simulink model "CRITIS_1_full"  (R2022b)
settings: Solver=VariableStepAuto  StartTime=0.0  StopTime=7  RelTol=1e-3
(part 2 of 13)

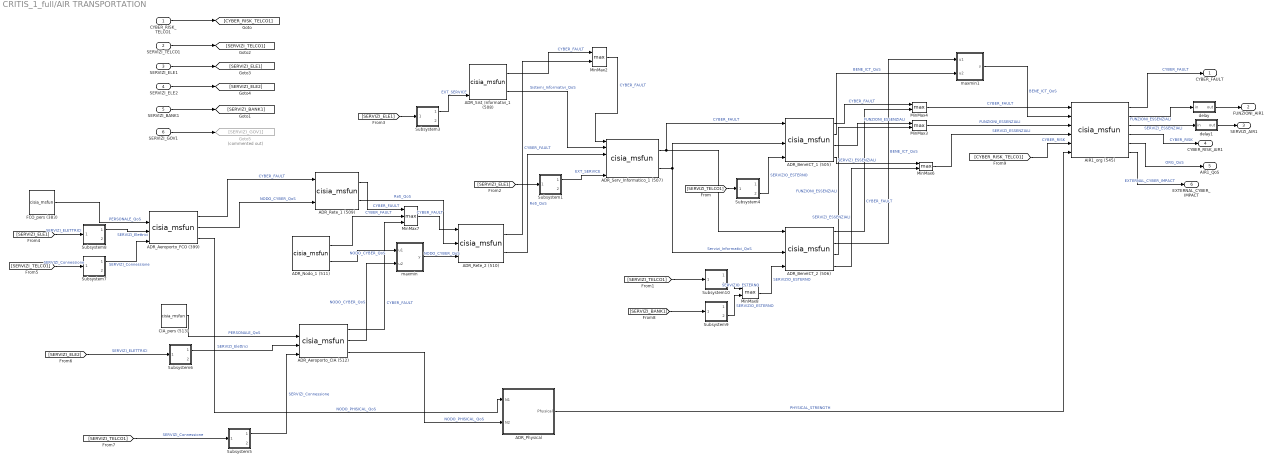
== system CRITIS_1_full/AIR TRANSPORTATION ==
  CYBER_RISK_TELCO1 : Inport
  SERVIZI_TELCO1 : Inport  Port=2
  SERVIZI_ELE1 : Inport  Port=3
  SERVIZI_ELE2 : Inport  Port=4
  SERVIZI_BANK1 : Inport  Port=5
  SERVIZI_GOV1 : Inport  Port=6
  ADR_Aeroporto_CIA (512) : M-S-Function  FunctionName=cisia_msfun  Parameters=Parameter1, Parameter2, Parameter3, resources, Parameter10, codeupdate, step_received, step_computed, dynamic_computed, step_sended, id_entity, id_project, id_type, name_type, color  mask(S-function:msfcn_unit_delay){Parameter1='ADR_Aeroporto_CIA', Parameter2=1, Parameter3='Iside', resources=|, Parameter10=off, codeupdate=off, step_received=|, step_computed=, dynamic_computed=, step_sended=|, id_entity=512, id_project=14, id_type=98, name_type=Nodo_Aeroporto, color=#FFFFFF}
      mask resources=|
      | *** INPUT RESOURCES ***
      | NUM_INPUTS 4
      | CYBER_FAULT (25)
      | PERSONALE_QoS (1)
      | SERVIZI_Elettrici (1)
      | SERVIZI_Connessione (1)
      |
      | *** STATE VARIABLES ***
      | NUM_VARIABLES 38
      | Operative_Level(NUMERIC)(1)(1)
      | Dos_attack(NUMERIC)(1)(0)
      | MITM_attack(NUMERIC)(1)(0)
      | Virus_Attack(NUMERIC)(1)(0)
      | Port_Scan_Attack(NUMERIC)(1)(0)
      | Cyber_Fault(NUMERIC_ARRAY)(25)(0  0  0  0  0  0  0  0  0  0  0  0  0  0  0  0  0  0  0  0  0  0  0  0  0)
      | BGP_hijacking(NUMERIC)(1)(0)
      | Mechanical_Fault(NUMERIC)(1)(0)
      | Power_Fault(NUMERIC)(1)(0)
      | Flooding_Fault(NUMERIC)(1)(0)
      | Fire_Fault(NUMERIC)(1)(0)
      | Unauthorized_Access(NUMERIC)(1)(0)
      | Conn_Fault(NUMERIC)(1)(0)
      | Service_Fault(NUMERIC)(1)(0)
      | BotNet_Attack(NUMERIC)(1)(0)
      | Data_Corruption(NUMERIC)(1)(0)
      | Rouge_Access(NUMERIC)(1)(0)
      | syslog_adm_login(NUMERIC)(1)(0)
      | SW_Change(NUMERIC)(1)(0)
      | Config_Change(NUMERIC)(1)(0)
      | Port_Saturation(NUMERIC)(1)(0)
      | Congestion_Fault(NUMERIC)(1)(0)
      | Perimeter_Security_Fault(NUMERIC)(1)(0)
      | Earthquake_Fault(NUMERIC)(1)(0)
      | Physical_Fault(NUMERIC)(1)(0)
      | Route_Poisoning(NUMERIC)(1)(0)
      | Interface_Down(NUMERIC)(1)(0)
      | Port_Isolation(NUMERIC)(1)(0)
      | Unknown_Device(NUMERIC)(1)(0)
      | USB_Device_Insertion(NUMERIC)(1)(0)
      | TLC_Fault(NUMERIC)(1)(0)
      | SW_Fault(NUMERIC)(1)(0)
      | Internal_Cyber_Risk(NUMERIC)(1)(0)
      | Data_Breach(NUMERIC)(1)(0)
      | Ransomware(NUMERIC)(1)(0)
      | Op_Level2(NUMERIC_ARRAY)(2)(0  0)
      | Possibility_Value(NUMERIC)(1)(0)
      | Necessity_Value(NUMERIC)(1)(0)
      |
      | *** OUTPUT RESOURCES ***
      | NUM_OUTPUTS 3
      | CYBER_FAULT (25)
      | NODO_CYBER_QoS (2)
      | NODO_PHISICAL_QoS (1)
      mask step_received=|
      | cyber_event=zeros(1,25);
      | cyber_event(1)=Dos_attack;
      | cyber_event(2)=MITM_attack;
      | cyber_event(3)=Virus_Attack;
      | cyber_event(4)=Port_Scan_Attack;
      | cyber_event(5)=BGP_hijacking;
      | cyber_event(6)=BotNet_Attack;
      | cyber_event(7)=Data_Corruption;
      | cyber_event(8)=SW_Change;
      | cyber_event(9)=Config_Change;
      | cyber_event(10)=Port_Saturation;
      | cyber_event(11)=Data_Breach;
      | cyber_event(12)=Unauthorized_Access;
      | cyber_event(13)=Unknown_Device;
      | cyber_event(14)=Congestion_Fault;
      | cyber_event(15)=Interface_Down;
      | cyber_event(16)=Port_Isolation;
      | cyber_event(17)=Rouge_Access;
      | cyber_event(18)=Route_Poisoning;
      | cyber_event(19)=SW_Fault;
      | cyber_event(20)=syslog_adm_login;
      | cyber_event(21)=USB_Device_Insertion;
      | cyber_event(22)=Ransomware;
      | cyber_event(23)=0;
      | cyber_event(24)=0;
      | cyber_event(25)=0;
      |
      | Cyber_Fault=max(CYBER_FAULT, transpose(cyber_event));
      |
      | TLC_Fault = 1 - SERVIZI_Connessione;
      | Power_Fault = 1-SERVIZI_Elettrici;
      |
      | Physical_Fault = max([Earthquake_Fault Fire_Fault Flooding_Fault Mechanical_Fault]);
      | Service_Fault = 1 - PERSONALE_QoS;
      |
      | Conn_Fault=max([(1-SERVIZI_Elettrici) (1-SERVIZI_Connessione)]);
      |
      | Operative_Level = (1-TLC_Fault)*(1-max(Cyber_Fault)*0.5)*(1-Physical_Fault)*(1-Power_Fault)*(1-Service_Fault);
      |
      | % Il primo elemento rappersenta possibility e si combima
      | % con il max in quanto rende conto del caso migliore
      | % (perche OL)
      |
      | Op_Level2(1)=  min([1-0.3*max(Cyber_Fault) 1-TLC_Fault 1-Power_Fault 1-Physical_Fault 1-Service_Fault]);
      |
      | % Il secondo elemento rappersenta necessity e si combima
      | % con il min in quanto rende conto del caso peggiore
      | % (perche OL)
      |
      | Op_Level2(2)= min([1-0.6*max(Cyber_Fault) 1-TLC_Fault 1-Power_Fault 1-Physical_Fault 1-Service_Fault]);
      |
      | Possibility_Value = Op_Level2(1);
      | Necessity_Value = Op_Level2(2);
      mask step_sended=|
      | CYBER_FAULT = Cyber_Fault;
      | % NODO_CYBER_QoS=(1-max(Cyber_Fault))*(1-Conn_Fault*0.5);
      | NODO_CYBER_QoS = Op_Level2;
      | NODO_PHISICAL_QoS=1-Physical_Fault;
      mask prompts: Parameter1 "entity name"; Parameter2 "sampling time"; Parameter3 "project"; resources "input resources and state variables"; Parameter10 "Bring state variables to output"; codeupdate "update code from mask"
      mask help: This is a level-2 MATLAB file S-function which demonstrates CISIA entity
      mask DialogControl Container1 Prompt: All parameters
      mask Display: disp('Nodo_Aeroporto');port_label('input',1,'\color{yellow}\spadesuit','texmode','on')
  ADR_Aeroporto_FCO (399) : M-S-Function  FunctionName=cisia_msfun  Parameters=Parameter1, Parameter2, Parameter3, resources, Parameter10, codeupdate, step_received, step_computed, dynamic_computed, step_sended, id_entity, id_project, id_type, name_type, color  mask(S-function:msfcn_unit_delay){Parameter1='ADR_Aeroporto_FCO', Parameter2=1, Parameter3='Iside', resources=|, Parameter10=off, codeupdate=off, step_received=|, step_computed=, dynamic_computed=, step_sended=|, id_entity=399, id_project=14, id_type=98, name_type=Nodo_Aeroporto, color=#FFFFFF}
      mask resources=|
      | *** INPUT RESOURCES ***
      | NUM_INPUTS 4
      | CYBER_FAULT (25)
      | PERSONALE_QoS (1)
      | SERVIZI_Elettrici (1)
      | SERVIZI_Connessione (1)
      |
      | *** STATE VARIABLES ***
      | NUM_VARIABLES 38
      | Operative_Level(NUMERIC)(1)(1)
      | Dos_attack(NUMERIC)(1)(0)
      | MITM_attack(NUMERIC)(1)(0)
      | Virus_Attack(NUMERIC)(1)(0)
      | Port_Scan_Attack(NUMERIC)(1)(0)
      | Cyber_Fault(NUMERIC_ARRAY)(25)(0  0  0  0  0  0  0  0  0  0  0  0  0  0  0  0  0  0  0  0  0  0  0  0  0)
      | BGP_hijacking(NUMERIC)(1)(0)
      | Mechanical_Fault(NUMERIC)(1)(0)
      | Power_Fault(NUMERIC)(1)(0)
      | Flooding_Fault(NUMERIC)(1)(0)
      | Fire_Fault(NUMERIC)(1)(0)
      | Unauthorized_Access(NUMERIC)(1)(0)
      | Conn_Fault(NUMERIC)(1)(0)
      | Service_Fault(NUMERIC)(1)(0)
      | BotNet_Attack(NUMERIC)(1)(0)
      | Data_Corruption(NUMERIC)(1)(0)
      | Rouge_Access(NUMERIC)(1)(0)
      | syslog_adm_login(NUMERIC)(1)(0)
      | SW_Change(NUMERIC)(1)(0)
      | Config_Change(NUMERIC)(1)(0)
      | Port_Saturation(NUMERIC)(1)(0)
      | Congestion_Fault(NUMERIC)(1)(0)
      | Perimeter_Security_Fault(NUMERIC)(1)(0)
      | Earthquake_Fault(NUMERIC)(1)(0)
      | Physical_Fault(NUMERIC)(1)(0)
      | Route_Poisoning(NUMERIC)(1)(0)
      | Interface_Down(NUMERIC)(1)(0)
      | Port_Isolation(NUMERIC)(1)(0)
      | Unknown_Device(NUMERIC)(1)(0)
      | USB_Device_Insertion(NUMERIC)(1)(0)
      | TLC_Fault(NUMERIC)(1)(0)
      | SW_Fault(NUMERIC)(1)(0)
      | Internal_Cyber_Risk(NUMERIC)(1)(0)
      | Data_Breach(NUMERIC)(1)(0)
      | Ransomware(NUMERIC)(1)(0)
      | Op_Level2(NUMERIC_ARRAY)(2)(0  0)
      | Possibility_Value(NUMERIC)(1)(0)
      | Necessity_Value(NUMERIC)(1)(0)
      |
      | *** OUTPUT RESOURCES ***
      | NUM_OUTPUTS 3
      | CYBER_FAULT (25)
      | NODO_CYBER_QoS (2)
      | NODO_PHISICAL_QoS (1)
      mask step_received=|
      | cyber_event=zeros(1,25);
      | cyber_event(1)=Dos_attack;
      | cyber_event(2)=MITM_attack;
      | cyber_event(3)=Virus_Attack;
      | cyber_event(4)=Port_Scan_Attack;
      | cyber_event(5)=BGP_hijacking;
      | cyber_event(6)=BotNet_Attack;
      | cyber_event(7)=Data_Corruption;
      | cyber_event(8)=SW_Change;
      | cyber_event(9)=Config_Change;
      | cyber_event(10)=Port_Saturation;
      | cyber_event(11)=Data_Breach;
      | cyber_event(12)=Unauthorized_Access;
      | cyber_event(13)=Unknown_Device;
      | cyber_event(14)=Congestion_Fault;
      | cyber_event(15)=Interface_Down;
      | cyber_event(16)=Port_Isolation;
      | cyber_event(17)=Rouge_Access;
      | cyber_event(18)=Route_Poisoning;
      | cyber_event(19)=SW_Fault;
      | cyber_event(20)=syslog_adm_login;
      | cyber_event(21)=USB_Device_Insertion;
      | cyber_event(22)=Ransomware;
      | cyber_event(23)=0;
      | cyber_event(24)=0;
      | cyber_event(25)=0;
      |
      | Cyber_Fault=max(CYBER_FAULT, transpose(cyber_event));
      |
      | TLC_Fault = 1 - SERVIZI_Connessione;
      | Power_Fault = 1-SERVIZI_Elettrici;
      |
      | Physical_Fault = max([Earthquake_Fault Fire_Fault Flooding_Fault Mechanical_Fault]);
      | Service_Fault = 1 - PERSONALE_QoS;
      |
      | Conn_Fault=max([(1-SERVIZI_Elettrici) (1-SERVIZI_Connessione)]);
      |
      | Operative_Level = (1-TLC_Fault)*(1-max(Cyber_Fault)*0.5)*(1-Physical_Fault)*(1-Power_Fault)*(1-Service_Fault);
      |
      | % Il primo elemento rappersenta possibility e si combima
      | % con il max in quanto rende conto del caso migliore
      | % (perche OL)
      |
      | Op_Level2(1)=  min([1-0.3*max(Cyber_Fault) 1-TLC_Fault 1-Power_Fault 1-Physical_Fault 1-Service_Fault]);
      |
      | % Il secondo elemento rappersenta necessity e si combima
      | % con il min in quanto rende conto del caso peggiore
      | % (perche OL)
      |
      | Op_Level2(2)= min([1-0.6*max(Cyber_Fault) 1-TLC_Fault 1-Power_Fault 1-Physical_Fault 1-Service_Fault]);
      |
      | Possibility_Value = Op_Level2(1);
      | Necessity_Value = Op_Level2(2);
      mask step_sended=|
      | CYBER_FAULT = Cyber_Fault;
      | % NODO_CYBER_QoS=(1-max(Cyber_Fault))*(1-Conn_Fault*0.5);
      | NODO_CYBER_QoS = Op_Level2;
      | NODO_PHISICAL_QoS=1-Physical_Fault;
      mask prompts: Parameter1 "entity name"; Parameter2 "sampling time"; Parameter3 "project"; resources "input resources and state variables"; Parameter10 "Bring state variables to output"; codeupdate "update code from mask"
      mask help: This is a level-2 MATLAB file S-function which demonstrates CISIA entity
      mask DialogControl Container1 Prompt: All parameters
      mask Display: disp('Nodo_Aeroporto');port_label('input',1,'\color{yellow}\spadesuit','texmode','on')
  ADR_BeneICT_1 (505) : M-S-Function  FunctionName=cisia_msfun  Parameters=Parameter1, Parameter2, Parameter3, resources, Parameter10, codeupdate, step_received, step_computed, dynamic_computed, step_sended, id_entity, id_project, id_type, name_type, color  mask(S-function:msfcn_unit_delay){Parameter1='ADR_BeneICT_1', Parameter2=1, Parameter3='Iside', resources=|, Parameter10=off, codeupdate=off, step_received=|, step_computed=, dynamic_computed=, step_sended=|, id_entity=505, id_project=14, id_type=108, name_type=BeneICT, color=#64D413}
      mask resources=|
      | *** INPUT RESOURCES ***
      | NUM_INPUTS 6
      | CYBER_FAULT (25)
      | Sistemi_Informativi_QoS (2)
      | Reti_QoS (2)
      | Servizi_Informatici_QoS (2)
      | BENE_ICT_QoS (2)
      | SERVIZIO_ESTERNO (20)
      |
      | *** STATE VARIABLES ***
      | NUM_VARIABLES 34
      | Operative_Level(NUMERIC)(1)(1)
      | Dos_attack(NUMERIC)(1)(0)
      | MITM_attack(NUMERIC)(1)(0)
      | Virus_Attack(NUMERIC)(1)(0)
      | Port_Scan_Attack(NUMERIC)(1)(0)
      | Cyber_Fault(NUMERIC_ARRAY)(25)(0  0  0  0  0  0  0  0  0  0  0  0  0  0  0  0  0  0  0  0  0  0  0  0  0)
      | BGP_hijacking(NUMERIC)(1)(0)
      | Unauthorized_Access(NUMERIC)(1)(0)
      | Consumed_Services(NUMERIC_ARRAY)(10)(0  0  0  0  0  0  0  0  0  0)
      | Service_Fault(NUMERIC)(1)(0)
      | BotNet_Attack(NUMERIC)(1)(0)
      | Data_Corruption(NUMERIC)(1)(0)
      | Rouge_Access(NUMERIC)(1)(0)
      | syslog_adm_login(NUMERIC)(1)(0)
      | SW_Change(NUMERIC)(1)(0)
      | Config_Change(NUMERIC)(1)(0)
      | Port_Saturation(NUMERIC)(1)(0)
      | Congestion_Fault(NUMERIC)(1)(0)
      | Route_Poisoning(NUMERIC)(1)(0)
      | Interface_Down(NUMERIC)(1)(0)
      | Port_Isolation(NUMERIC)(1)(0)
      | Unknown_Device(NUMERIC)(1)(0)
      | USB_Device_Insertion(NUMERIC)(1)(0)
      | SW_Fault(NUMERIC)(1)(0)
      | Servizi_Essenziali(NUMERIC_ARRAY)(10)(1  0  0  0  0  0  0  0  0  0)
      | Funzioni_Essenziali(NUMERIC_ARRAY)(10)(0  0  0  0  0  0  0  0  0  0)
      | Consumed_Functions(NUMERIC_ARRAY)(10)(0  0  0  0  0  0  0  0  0  0)
      | Internal_Cyber_Risk(NUMERIC)(1)(0)
      | Data_Breach(NUMERIC)(1)(0)
      | availability_fault(NUMERIC)(1)(0)
      | Ransomware(NUMERIC)(1)(0)
      | Op_Level2(NUMERIC_ARRAY)(2)(0  0)
      | Possibility_Value(NUMERIC)(1)(0)
      | Necessity_Value(NUMERIC)(1)(0)
      |
      | *** OUTPUT RESOURCES ***
      | NUM_OUTPUTS 4
      | CYBER_FAULT (25)
      | BENE_ICT_QoS (2)
      | FUNZIONI_ESSENZIALI (10)
      | SERVIZI_ESSENZIALI (10)
      mask step_received=|
      | cyber_event=zeros(1,25);
      | cyber_event(1)=Dos_attack;
      | cyber_event(2)=MITM_attack;
      | cyber_event(3)=Virus_Attack;
      | cyber_event(4)=Port_Scan_Attack;
      | cyber_event(5)=BGP_hijacking;
      | cyber_event(6)=BotNet_Attack;
      | cyber_event(7)=Data_Corruption;
      | cyber_event(8)=SW_Change;
      | cyber_event(9)=Config_Change;
      | cyber_event(10)=Port_Saturation;
      | cyber_event(11)=Data_Breach;
      | cyber_event(12)=Unauthorized_Access;
      | cyber_event(13)=Unknown_Device;
      | cyber_event(14)=Congestion_Fault;
      | cyber_event(15)=Interface_Down;
      | cyber_event(16)=Port_Isolation;
      | cyber_event(17)=Rouge_Access;
      | cyber_event(18)=Route_Poisoning;
      | cyber_event(19)=SW_Fault;
      | cyber_event(20)=syslog_adm_login;
      | cyber_event(21)=USB_Device_Insertion;
      | cyber_event(22)=Ransomware;
      | cyber_event(23)=0;
      | cyber_event(24)=0;
      | cyber_event(25)=0;
      |
      | Cyber_Fault=max(CYBER_FAULT, transpose(cyber_event));
      |
      | Consumed_Services=SERVIZIO_ESTERNO(1:10);
      | Consumed_Functions=SERVIZIO_ESTERNO(11:20);
      |
      | Service_Fault=max(abs(Servizi_Essenziali-Consumed_Services));
      |
      | availability_fault=1-min([(1-0.5*max(Cyber_Fault)) min(Reti_QoS) min(Sistemi_Informativi_QoS) min(Servizi_Informatici_QoS) min(BENE_ICT_QoS)]);
      |
      | Operative_Level=min([(1-0.5*max(Cyber_Fault)) mean(Reti_QoS) mean(Sistemi_Informativi_QoS) mean(Servizi_Informatici_QoS) mean(BENE_ICT_QoS) 1-Service_Fault]);
      |
      | % Il primo elemento rappersenta possibility e si combima
      | % con il max in quanto rende conto del caso migliore
      | % (perche OL)
      |
      | BNICT=BENE_ICT_QoS;
      |
      | Op_Level2(1)=  min([1-0.3*max(Cyber_Fault) max([use_elem(Reti_QoS,1) use_elem(Sistemi_Informativi_QoS,1) use_elem(Servizi_Informatici_QoS,1) use_elem(BENE_ICT_QoS,1)]) 1-Service_Fault]);
      |
      | % Il secondo elemento rappresenta necessity e si combima
      | % con il min in quanto rende conto del caso peggiore
      | % (perche OL)
      |
      |
      |
      | Op_Level2(2)= min([1-0.6*max(Cyber_Fault) min([use_elem(Reti_QoS,2) use_elem(Sistemi_Informativi_QoS,2) use_elem(Servizi_Informatici_QoS,2) use_elem(BENE_ICT_QoS,2)]) 1-Service_Fault]);
      |
      | Possibility_Value = Op_Level2(1);
      | Necessity_Value = Op_Level2(2);
      mask step_sended=|
      | CYBER_FAULT=Cyber_Fault;
      |
      | FUNZIONI_ESSENZIALI=(1-availability_fault)*Funzioni_Essenziali.*Consumed_Functions;
      |
      | SERVIZI_ESSENZIALI=(1-availability_fault)*Servizi_Essenziali.*Consumed_Services;
      |
      | BENE_ICT_QoS=Op_Level2;
      mask prompts: Parameter1 "entity name"; Parameter2 "sampling time"; Parameter3 "project"; resources "input resources and state variables"; Parameter10 "Bring state variables to output"; codeupdate "update code from mask"
      mask help: This is a level-2 MATLAB file S-function which demonstrates CISIA entity
      mask DialogControl Container1 Prompt: All parameters
      mask Display: disp('BeneICT');port_label('input',2,'\color{yellow}\spadesuit','texmode','on');port_label('input',3,'\color{yellow}\spadesuit','texmode','on');port_label('input',5,'\color{yellow}\spadesuit','texmode','on')
  ADR_BeneICT_2 (506) : M-S-Function  FunctionName=cisia_msfun  Parameters=Parameter1, Parameter2, Parameter3, resources, Parameter10, codeupdate, step_received, step_computed, dynamic_computed, step_sended, id_entity, id_project, id_type, name_type, color  mask(S-function:msfcn_unit_delay){Parameter1='ADR_BeneICT_2', Parameter2=1, Parameter3='Iside', resources=|, Parameter10=off, codeupdate=off, step_received=|, step_computed=, dynamic_computed=, step_sended=|, id_entity=506, id_project=14, id_type=108, name_type=BeneICT, color=#64D413}
      mask resources=|
      | *** INPUT RESOURCES ***
      | NUM_INPUTS 6
      | CYBER_FAULT (25)
      | Sistemi_Informativi_QoS (2)
      | Reti_QoS (2)
      | Servizi_Informatici_QoS (2)
      | BENE_ICT_QoS (2)
      | SERVIZIO_ESTERNO (20)
      |
      | *** STATE VARIABLES ***
      | NUM_VARIABLES 34
      | Operative_Level(NUMERIC)(1)(1)
      | Dos_attack(NUMERIC)(1)(0)
      | MITM_attack(NUMERIC)(1)(0)
      | Virus_Attack(NUMERIC)(1)(0)
      | Port_Scan_Attack(NUMERIC)(1)(0)
      | Cyber_Fault(NUMERIC_ARRAY)(25)(0  0  0  0  0  0  0  0  0  0  0  0  0  0  0  0  0  0  0  0  0  0  0  0  0)
      | BGP_hijacking(NUMERIC)(1)(0)
      | Unauthorized_Access(NUMERIC)(1)(0)
      | Consumed_Services(NUMERIC_ARRAY)(10)(0  0  0  0  0  0  0  0  0  0)
      | Service_Fault(NUMERIC)(1)(0)
      | BotNet_Attack(NUMERIC)(1)(0)
      | Data_Corruption(NUMERIC)(1)(0)
      | Rouge_Access(NUMERIC)(1)(0)
      | syslog_adm_login(NUMERIC)(1)(0)
      | SW_Change(NUMERIC)(1)(0)
      | Config_Change(NUMERIC)(1)(0)
      | Port_Saturation(NUMERIC)(1)(0)
      | Congestion_Fault(NUMERIC)(1)(0)
      | Route_Poisoning(NUMERIC)(1)(0)
      | Interface_Down(NUMERIC)(1)(0)
      | Port_Isolation(NUMERIC)(1)(0)
      | Unknown_Device(NUMERIC)(1)(0)
      | USB_Device_Insertion(NUMERIC)(1)(0)
      | SW_Fault(NUMERIC)(1)(0)
      | Servizi_Essenziali(NUMERIC_ARRAY)(10)(0  1  1  0  0  0  0  0  0  0)
      | Funzioni_Essenziali(NUMERIC_ARRAY)(10)(0  0  0  0  0  0  0  0  0  0)
      | Consumed_Functions(NUMERIC_ARRAY)(10)(0  0  0  0  0  0  0  0  0  0)
      | Internal_Cyber_Risk(NUMERIC)(1)(0)
      | Data_Breach(NUMERIC)(1)(0)
      | availability_fault(NUMERIC)(1)(0)
      | Ransomware(NUMERIC)(1)(0)
      | Op_Level2(NUMERIC_ARRAY)(2)(0  0)
      | Possibility_Value(NUMERIC)(1)(0)
      | Necessity_Value(NUMERIC)(1)(0)
      |
      | *** OUTPUT RESOURCES ***
      | NUM_OUTPUTS 4
      | CYBER_FAULT (25)
      | BENE_ICT_QoS (2)
      | FUNZIONI_ESSENZIALI (10)
      | SERVIZI_ESSENZIALI (10)
      mask step_received=|
      | cyber_event=zeros(1,25);
      | cyber_event(1)=Dos_attack;
      | cyber_event(2)=MITM_attack;
      | cyber_event(3)=Virus_Attack;
      | cyber_event(4)=Port_Scan_Attack;
      | cyber_event(5)=BGP_hijacking;
      | cyber_event(6)=BotNet_Attack;
      | cyber_event(7)=Data_Corruption;
      | cyber_event(8)=SW_Change;
      | cyber_event(9)=Config_Change;
      | cyber_event(10)=Port_Saturation;
      | cyber_event(11)=Data_Breach;
      | cyber_event(12)=Unauthorized_Access;
      | cyber_event(13)=Unknown_Device;
      | cyber_event(14)=Congestion_Fault;
      | cyber_event(15)=Interface_Down;
      | cyber_event(16)=Port_Isolation;
      | cyber_event(17)=Rouge_Access;
      | cyber_event(18)=Route_Poisoning;
      | cyber_event(19)=SW_Fault;
      | cyber_event(20)=syslog_adm_login;
      | cyber_event(21)=USB_Device_Insertion;
      | cyber_event(22)=Ransomware;
      | cyber_event(23)=0;
      | cyber_event(24)=0;
      | cyber_event(25)=0;
      |
      | Cyber_Fault=max(CYBER_FAULT, transpose(cyber_event));
      |
      | Consumed_Services=SERVIZIO_ESTERNO(1:10);
      | Consumed_Functions=SERVIZIO_ESTERNO(11:20);
      |
      | Service_Fault=max(abs(Servizi_Essenziali-Consumed_Services));
      |
      | availability_fault=1-min([(1-0.5*max(Cyber_Fault)) min(Reti_QoS) min(Sistemi_Informativi_QoS) min(Servizi_Informatici_QoS) min(BENE_ICT_QoS)]);
      |
      | Operative_Level=min([(1-0.5*max(Cyber_Fault)) mean(Reti_QoS) mean(Sistemi_Informativi_QoS) mean(Servizi_Informatici_QoS) mean(BENE_ICT_QoS) 1-Service_Fault]);
      |
      | % Il primo elemento rappersenta possibility e si combima
      | % con il max in quanto rende conto del caso migliore
      | % (perche OL)
      |
      | BNICT=BENE_ICT_QoS;
      |
      | Op_Level2(1)=  min([1-0.3*max(Cyber_Fault) max([use_elem(Reti_QoS,1) use_elem(Sistemi_Informativi_QoS,1) use_elem(Servizi_Informatici_QoS,1) use_elem(BENE_ICT_QoS,1)]) 1-Service_Fault]);
      |
      | % Il secondo elemento rappresenta necessity e si combima
      | % con il min in quanto rende conto del caso peggiore
      | % (perche OL)
      |
      |
      |
      | Op_Level2(2)= min([1-0.6*max(Cyber_Fault) min([use_elem(Reti_QoS,2) use_elem(Sistemi_Informativi_QoS,2) use_elem(Servizi_Informatici_QoS,2) use_elem(BENE_ICT_QoS,2)]) 1-Service_Fault]);
      |
      | Possibility_Value = Op_Level2(1);
      | Necessity_Value = Op_Level2(2);
      mask step_sended=|
      | CYBER_FAULT=Cyber_Fault;
      |
      | FUNZIONI_ESSENZIALI=(1-availability_fault)*Funzioni_Essenziali.*Consumed_Functions;
      |
      | SERVIZI_ESSENZIALI=(1-availability_fault)*Servizi_Essenziali.*Consumed_Services;
      |
      | BENE_ICT_QoS=Op_Level2;
      mask prompts: Parameter1 "entity name"; Parameter2 "sampling time"; Parameter3 "project"; resources "input resources and state variables"; Parameter10 "Bring state variables to output"; codeupdate "update code from mask"
      mask help: This is a level-2 MATLAB file S-function which demonstrates CISIA entity
      mask DialogControl Container1 Prompt: All parameters
      mask Display: disp('BeneICT');port_label('input',2,'\color{yellow}\spadesuit','texmode','on');port_label('input',3,'\color{yellow}\spadesuit','texmode','on');port_label('input',5,'\color{yellow}\spadesuit','texmode','on')
  ADR_Nodo_1 (511) : M-S-Function  FunctionName=cisia_msfun  Parameters=Parameter1, Parameter2, Parameter3, resources, Parameter10, codeupdate, step_received, step_computed, dynamic_computed, step_sended, id_entity, id_project, id_type, name_type, color  mask(S-function:msfcn_unit_delay){Parameter1='ADR_Nodo_1', Parameter2=1, Parameter3='Iside', resources=|, Parameter10=off, codeupdate=off, step_received=|, step_computed=, dynamic_computed=, step_sended=|, id_entity=511, id_project=14, id_type=109, name_type=Nodo_Datacenter, color=#DCF6F7}
      mask resources=|
      | *** INPUT RESOURCES ***
      | NUM_INPUTS 0
      |
      | *** STATE VARIABLES ***
      | NUM_VARIABLES 32
      | Operative_Level(NUMERIC)(1)(1)
      | Dos_attack(NUMERIC)(1)(0)
      | MITM_attack(NUMERIC)(1)(0)
      | Virus_Attack(NUMERIC)(1)(0)
      | Port_Scan_Attack(NUMERIC)(1)(0)
      | Cyber_Fault(NUMERIC_ARRAY)(25)(0  0  0  0  0  0  0  0  0  0  0  0  0  0  0  0  0  0  0  0  0  0  0  0  0)
      | BGP_hijacking(NUMERIC)(1)(0)
      | Mechanical_Fault(NUMERIC)(1)(0)
      | Unauthorized_Access(NUMERIC)(1)(0)
      | Conn_Fault(NUMERIC)(1)(0)
      | BotNet_Attack(NUMERIC)(1)(0)
      | Data_Corruption(NUMERIC)(1)(0)
      | Rouge_Access(NUMERIC)(1)(0)
      | syslog_adm_login(NUMERIC)(1)(0)
      | SW_Change(NUMERIC)(1)(0)
      | Config_Change(NUMERIC)(1)(0)
      | Port_Saturation(NUMERIC)(1)(0)
      | Congestion_Fault(NUMERIC)(1)(0)
      | Route2(NUMERIC)(1)(0)
      | Route_Poisoning(NUMERIC)(1)(0)
      | Interface_Down(NUMERIC)(1)(0)
      | Port_Isolation(NUMERIC)(1)(0)
      | Unknown_Device(NUMERIC)(1)(0)
      | USB_Device_Insertion(NUMERIC)(1)(0)
      | GEO_localization(STRING)(100)()
      | SW_Fault(NUMERIC)(1)(0)
      | Internal_Cyber_Risk(NUMERIC)(1)(0)
      | Data_Breach(NUMERIC)(1)(0)
      | Ransomware(NUMERIC)(1)(0)
      | Op_Level2(NUMERIC_ARRAY)(2)(0  0)
      | Possibility_Value(NUMERIC)(1)(0)
      | Necessity_Value(NUMERIC)(1)(0)
      |
      | *** OUTPUT RESOURCES ***
      | NUM_OUTPUTS 2
      | CYBER_FAULT (25)
      | NODO_CYBER_QoS (2)
      mask step_received=|
      | cyber_event=zeros(1,25);
      | cyber_event(1)=Dos_attack;
      | cyber_event(2)=MITM_attack;
      | cyber_event(3)=Virus_Attack;
      | cyber_event(4)=Port_Scan_Attack;
      | cyber_event(5)=BGP_hijacking;
      | cyber_event(6)=BotNet_Attack;
      | cyber_event(7)=Data_Corruption;
      | cyber_event(8)=SW_Change;
      | cyber_event(9)=Config_Change;
      | cyber_event(10)=Port_Saturation;
      | cyber_event(11)=Data_Breach;
      | cyber_event(12)=Unauthorized_Access;
      | cyber_event(13)=Unknown_Device;
      | cyber_event(14)=Congestion_Fault;
      | cyber_event(15)=Interface_Down;
      | cyber_event(16)=Port_Isolation;
      | cyber_event(17)=Rouge_Access;
      | cyber_event(18)=Route_Poisoning;
      | cyber_event(19)=SW_Fault;
      | cyber_event(20)=syslog_adm_login;
      | cyber_event(21)=USB_Device_Insertion;
      | cyber_event(22)=Ransomware;
      | cyber_event(23)=0;
      | cyber_event(24)=0;
      | cyber_event(25)=0;
      |
      | Cyber_Fault=transpose(cyber_event);
      |
      | Conn_Fault=max([Dos_attack BGP_hijacking Route_Poisoning Interface_Down Mechanical_Fault] );
      |
      |
      | Operative_Level=min((1-Conn_Fault),(1-0.5*max(Cyber_Fault)));
      |
      | % Il primo elemento rappersenta possibility e si combima
      | % con il max in quanto rende conto del caso migliore
      | % (perche OL)
      |
      | Op_Level2(1)=  min([1-0.3*max(Cyber_Fault) 1-Conn_Fault]);
      |
      | % Il secondo elemento rappersenta necessity e si combima
      | % con il min in quanto rende conto del caso peggiore
      | % (perche OL)
      |
      | Op_Level2(2)= min([1-0.6*max(Cyber_Fault) 1-Conn_Fault]);
      |
      | Possibility_Value = Op_Level2(1);
      | Necessity_Value = Op_Level2(2);
      mask step_sended=|
      | CYBER_FAULT=Cyber_Fault;
      |
      |
      | NODO_CYBER_QoS=Op_Level2;
      mask prompts: Parameter1 "entity name"; Parameter2 "sampling time"; Parameter3 "project"; resources "input resources and state variables"; Parameter10 "Bring state variables to output"; codeupdate "update code from mask"
      mask help: This is a level-2 MATLAB file S-function which demonstrates CISIA entity
      mask DialogControl Container1 Prompt: All parameters
      mask Display: disp('Nodo_Datacenter')
  ADR_Physical : MATLAB Function  TreatAsAtomicUnit=on
  ADR_Rete_1 (509) : M-S-Function  FunctionName=cisia_msfun  Parameters=Parameter1, Parameter2, Parameter3, resources, Parameter10, codeupdate, step_received, step_computed, dynamic_computed, step_sended, id_entity, id_project, id_type, name_type, color  mask(S-function:msfcn_unit_delay){Parameter1='ADR_Rete_1', Parameter2=1, Parameter3='Iside', resources=|, Parameter10=off, codeupdate=off, step_received=|, step_computed=, dynamic_computed=, step_sended=|, id_entity=509, id_project=14, id_type=82, name_type=Reti_Sito, color=#45B5ED}
      mask resources=|
      | *** INPUT RESOURCES ***
      | NUM_INPUTS 3
      | CYBER_FAULT (25)
      | Reti_QoS (2)
      | NODO_CYBER_QoS (2)
      |
      | *** STATE VARIABLES ***
      | NUM_VARIABLES 34
      | Operative_Level(NUMERIC)(1)(1)
      | Dos_attack(NUMERIC)(1)(0)
      | MITM_attack(NUMERIC)(1)(0)
      | Virus_Attack(NUMERIC)(1)(0)
      | Port_Scan_Attack(NUMERIC)(1)(0)
      | Cyber_Fault(NUMERIC_ARRAY)(25)(0  0  0  0  0  0  0  0  0  0  0  0  0  0  0  0  0  0  0  0  0  0  0  0  0)
      | BGP_hijacking(NUMERIC)(1)(0)
      | Mechanical_Fault(NUMERIC)(1)(0)
      | Unauthorized_Access(NUMERIC)(1)(0)
      | Conn_Fault(NUMERIC)(1)(0)
      | BotNet_Attack(NUMERIC)(1)(0)
      | Data_Corruption(NUMERIC)(1)(0)
      | Rouge_Access(NUMERIC)(1)(0)
      | syslog_adm_login(NUMERIC)(1)(0)
      | SW_Change(NUMERIC)(1)(0)
      | Config_Change(NUMERIC)(1)(0)
      | Port_Saturation(NUMERIC)(1)(0)
      | Congestion_Fault(NUMERIC)(1)(0)
      | Physical_Fault(NUMERIC)(1)(0)
      | Route2(NUMERIC)(1)(0)
      | Route_Poisoning(NUMERIC)(1)(0)
      | Interface_Down(NUMERIC)(1)(0)
      | Port_Isolation(NUMERIC)(1)(0)
      | Unknown_Device(NUMERIC)(1)(0)
      | USB_Device_Insertion(NUMERIC)(1)(0)
      | Risorsa(NUMERIC)(1)(0)
      | GEO_localization(STRING)(100)()
      | SW_Fault(NUMERIC)(1)(0)
      | Internal_Cyber_Risk(NUMERIC)(1)(0)
      | Data_Breach(NUMERIC)(1)(0)
      | Ransomware(NUMERIC)(1)(0)
      | Op_Level2(NUMERIC_ARRAY)(2)(0  0)
      | Possibility_Value(NUMERIC)(1)(0)
      | Necessity_Value(NUMERIC)(1)(0)
      |
      | *** OUTPUT RESOURCES ***
      | NUM_OUTPUTS 2
      | CYBER_FAULT (25)
      | Reti_QoS (2)
      mask step_received=|
      | cyber_event=zeros(1,25);
      | cyber_event(1)=Dos_attack;
      | cyber_event(2)=MITM_attack;
      | cyber_event(3)=Virus_Attack;
      | cyber_event(4)=Port_Scan_Attack;
      | cyber_event(5)=BGP_hijacking;
      | cyber_event(6)=BotNet_Attack;
      | cyber_event(7)=Data_Corruption;
      | cyber_event(8)=SW_Change;
      | cyber_event(9)=Config_Change;
      | cyber_event(10)=Port_Saturation;
      | cyber_event(11)=Data_Breach;
      | cyber_event(12)=Unauthorized_Access;
      | cyber_event(13)=Unknown_Device;
      | cyber_event(14)=Congestion_Fault;
      | cyber_event(15)=Interface_Down;
      | cyber_event(16)=Port_Isolation;
      | cyber_event(17)=Rouge_Access;
      | cyber_event(18)=Route_Poisoning;
      | cyber_event(19)=SW_Fault;
      | cyber_event(20)=syslog_adm_login;
      | cyber_event(21)=USB_Device_Insertion;
      | cyber_event(22)=Ransomware;
      | cyber_event(23)=0;
      | cyber_event(24)=0;
      | cyber_event(25)=0;
      |
      | Cyber_Fault=max(CYBER_FAULT, transpose(cyber_event));
      |
      | Conn_Fault=max([Dos_attack BGP_hijacking Route_Poisoning Interface_Down Mechanical_Fault] );
      |
      | Operative_Level=min([(1-Conn_Fault) (1-0.5*max(Cyber_Fault))  mean(Reti_QoS)  mean(NODO_CYBER_QoS)]);
      |
      | % Il primo elemento rappersenta possibility e si combima
      | % con il max in quanto rende conto del caso migliore
      | % (perche OL)
      |
      | Op_Level2(1)=  min([1-0.3*max(Cyber_Fault) max([use_elem(Reti_QoS,1) use_elem(NODO_CYBER_QoS,1)]) 1-Conn_Fault]);
      |
      | % Il secondo elemento rappersenta necessity e si combima
      | % con il min in quanto rende conto del caso peggiore
      | % (perche OL)
      |
      | Op_Level2(2)= min([1-0.6*max(Cyber_Fault) min([use_elem(Reti_QoS,2) use_elem(NODO_CYBER_QoS,2)]) 1-Conn_Fault]);
      |
      | Possibility_Value = Op_Level2(1);
      | Necessity_Value = Op_Level2(2);
      mask step_sended=|
      | CYBER_FAULT=Cyber_Fault;
      |
      |
      | Reti_QoS=Op_Level2;
      mask prompts: Parameter1 "entity name"; Parameter2 "sampling time"; Parameter3 "project"; resources "input resources and state variables"; Parameter10 "Bring state variables to output"; codeupdate "update code from mask"
      mask help: This is a level-2 MATLAB file S-function which demonstrates CISIA entity
      mask DialogControl Container1 Prompt: All parameters
      mask Display: disp('Reti_Sito');port_label('input',2,'\color{yellow}\spadesuit','texmode','on')
  ADR_Rete_2 (510) : M-S-Function  FunctionName=cisia_msfun  Parameters=Parameter1, Parameter2, Parameter3, resources, Parameter10, codeupdate, step_received, step_computed, dynamic_computed, step_sended, id_entity, id_project, id_type, name_type, color  mask(S-function:msfcn_unit_delay){Parameter1='ADR_Rete_2', Parameter2=1, Parameter3='Iside', resources=|, Parameter10=off, codeupdate=off, step_received=|, step_computed=, dynamic_computed=, step_sended=|, id_entity=510, id_project=14, id_type=82, name_type=Reti_Sito, color=#45B5ED}
      mask resources=|
      | *** INPUT RESOURCES ***
      | NUM_INPUTS 3
      | CYBER_FAULT (25)
      | Reti_QoS (2)
      | NODO_CYBER_QoS (2)
      |
      | *** STATE VARIABLES ***
      | NUM_VARIABLES 34
      | Operative_Level(NUMERIC)(1)(1)
      | Dos_attack(NUMERIC)(1)(0)
      | MITM_attack(NUMERIC)(1)(0)
      | Virus_Attack(NUMERIC)(1)(0)
      | Port_Scan_Attack(NUMERIC)(1)(0)
      | Cyber_Fault(NUMERIC_ARRAY)(25)(0  0  0  0  0  0  0  0  0  0  0  0  0  0  0  0  0  0  0  0  0  0  0  0  0)
      | BGP_hijacking(NUMERIC)(1)(0)
      | Mechanical_Fault(NUMERIC)(1)(0)
      | Unauthorized_Access(NUMERIC)(1)(0)
      | Conn_Fault(NUMERIC)(1)(0)
      | BotNet_Attack(NUMERIC)(1)(0)
      | Data_Corruption(NUMERIC)(1)(0)
      | Rouge_Access(NUMERIC)(1)(0)
      | syslog_adm_login(NUMERIC)(1)(0)
      | SW_Change(NUMERIC)(1)(0)
      | Config_Change(NUMERIC)(1)(0)
      | Port_Saturation(NUMERIC)(1)(0)
      | Congestion_Fault(NUMERIC)(1)(0)
      | Physical_Fault(NUMERIC)(1)(0)
      | Route2(NUMERIC)(1)(0)
      | Route_Poisoning(NUMERIC)(1)(0)
      | Interface_Down(NUMERIC)(1)(0)
      | Port_Isolation(NUMERIC)(1)(0)
      | Unknown_Device(NUMERIC)(1)(0)
      | USB_Device_Insertion(NUMERIC)(1)(0)
      | Risorsa(NUMERIC)(1)(0)
      | GEO_localization(STRING)(100)()
      | SW_Fault(NUMERIC)(1)(0)
      | Internal_Cyber_Risk(NUMERIC)(1)(0)
      | Data_Breach(NUMERIC)(1)(0)
      | Ransomware(NUMERIC)(1)(0)
      | Op_Level2(NUMERIC_ARRAY)(2)(0  0)
      | Possibility_Value(NUMERIC)(1)(0)
      | Necessity_Value(NUMERIC)(1)(0)
      |
      | *** OUTPUT RESOURCES ***
      | NUM_OUTPUTS 2
      | CYBER_FAULT (25)
      | Reti_QoS (2)
      mask step_received=|
      | cyber_event=zeros(1,25);
      | cyber_event(1)=Dos_attack;
      | cyber_event(2)=MITM_attack;
      | cyber_event(3)=Virus_Attack;
      | cyber_event(4)=Port_Scan_Attack;
      | cyber_event(5)=BGP_hijacking;
      | cyber_event(6)=BotNet_Attack;
      | cyber_event(7)=Data_Corruption;
      | cyber_event(8)=SW_Change;
      | cyber_event(9)=Config_Change;
      | cyber_event(10)=Port_Saturation;
      | cyber_event(11)=Data_Breach;
      | cyber_event(12)=Unauthorized_Access;
      | cyber_event(13)=Unknown_Device;
      | cyber_event(14)=Congestion_Fault;
      | cyber_event(15)=Interface_Down;
      | cyber_event(16)=Port_Isolation;
      | cyber_event(17)=Rouge_Access;
      | cyber_event(18)=Route_Poisoning;
      | cyber_event(19)=SW_Fault;
      | cyber_event(20)=syslog_adm_login;
      | cyber_event(21)=USB_Device_Insertion;
      | cyber_event(22)=Ransomware;
      | cyber_event(23)=0;
      | cyber_event(24)=0;
      | cyber_event(25)=0;
      |
      | Cyber_Fault=max(CYBER_FAULT, transpose(cyber_event));
      |
      | Conn_Fault=max([Dos_attack BGP_hijacking Route_Poisoning Interface_Down Mechanical_Fault] );
      |
      | Operative_Level=min([(1-Conn_Fault) (1-0.5*max(Cyber_Fault))  mean(Reti_QoS)  mean(NODO_CYBER_QoS)]);
      |
      | % Il primo elemento rappersenta possibility e si combima
      | % con il max in quanto rende conto del caso migliore
      | % (perche OL)
      |
      | Op_Level2(1)=  min([1-0.3*max(Cyber_Fault) max([use_elem(Reti_QoS,1) use_elem(NODO_CYBER_QoS,1)]) 1-Conn_Fault]);
      |
      | % Il secondo elemento rappersenta necessity e si combima
      | % con il min in quanto rende conto del caso peggiore
      | % (perche OL)
      |
      | Op_Level2(2)= min([1-0.6*max(Cyber_Fault) min([use_elem(Reti_QoS,2) use_elem(NODO_CYBER_QoS,2)]) 1-Conn_Fault]);
      |
      | Possibility_Value = Op_Level2(1);
      | Necessity_Value = Op_Level2(2);
      mask step_sended=|
      | CYBER_FAULT=Cyber_Fault;
      |
      |
      | Reti_QoS=Op_Level2;
      mask prompts: Parameter1 "entity name"; Parameter2 "sampling time"; Parameter3 "project"; resources "input resources and state variables"; Parameter10 "Bring state variables to output"; codeupdate "update code from mask"
      mask help: This is a level-2 MATLAB file S-function which demonstrates CISIA entity
      mask DialogControl Container1 Prompt: All parameters
      mask Display: disp('Reti_Sito')
  ADR_Serv_Informatico_1 (507) : M-S-Function  FunctionName=cisia_msfun  Parameters=Parameter1, Parameter2, Parameter3, resources, Parameter10, codeupdate, step_received, step_computed, dynamic_computed, step_sended, id_entity, id_project, id_type, name_type, color  mask(S-function:msfcn_unit_delay){Parameter1='ADR_Serv_Informatico_1', Parameter2=1, Parameter3='Iside', resources=|, Parameter10=off, codeupdate=off, step_received=|, step_computed=, dynamic_computed=, step_sended=|, id_entity=507, id_project=14, id_type=83, name_type=Servizi_Informatici, color=#6FD0E8}
      mask resources=|
      | *** INPUT RESOURCES ***
      | NUM_INPUTS 6
      | CYBER_FAULT (25)
      | Sistemi_Informativi_QoS (2)
      | Reti_QoS (2)
      | Servizi_Informatici_QoS (2)
      | BENE_ICT_QoS (2)
      | EXT_SERVICE (1)
      |
      | *** STATE VARIABLES ***
      | NUM_VARIABLES 31
      | Operative_Level(NUMERIC)(1)(1)
      | Dos_attack(NUMERIC)(1)(0)
      | MITM_attack(NUMERIC)(1)(0)
      | Virus_Attack(NUMERIC)(1)(0)
      | Port_Scan_Attack(NUMERIC)(1)(0)
      | Cyber_Fault(NUMERIC_ARRAY)(25)(0  0  0  0  0  0  0  0  0  0  0  0  0  0  0  0  0  0  0  0  0  0  0  0  0)
      | BGP_hijacking(NUMERIC)(1)(0)
      | Mechanical_Fault(NUMERIC)(1)(0)
      | Unauthorized_Access(NUMERIC)(1)(0)
      | Service_Fault(NUMERIC)(1)(0)
      | BotNet_Attack(NUMERIC)(1)(0)
      | Data_Corruption(NUMERIC)(1)(0)
      | Rouge_Access(NUMERIC)(1)(0)
      | syslog_adm_login(NUMERIC)(1)(0)
      | SW_Change(NUMERIC)(1)(0)
      | Config_Change(NUMERIC)(1)(0)
      | Port_Saturation(NUMERIC)(1)(0)
      | Congestion_Fault(NUMERIC)(1)(0)
      | Route2(NUMERIC)(1)(0)
      | Route_Poisoning(NUMERIC)(1)(0)
      | Interface_Down(NUMERIC)(1)(0)
      | Port_Isolation(NUMERIC)(1)(0)
      | Unknown_Device(NUMERIC)(1)(0)
      | USB_Device_Insertion(NUMERIC)(1)(0)
      | SW_Fault(NUMERIC)(1)(0)
      | Internal_Cyber_Risk(NUMERIC)(1)(0)
      | Data_Breach(NUMERIC)(1)(0)
      | Ransomware(NUMERIC)(1)(0)
      | Op_Level2(NUMERIC_ARRAY)(2)(0  0)
      | Possibility_Value(NUMERIC)(1)(0)
      | Necessity_Value(NUMERIC)(1)(0)
      |
      | *** OUTPUT RESOURCES ***
      | NUM_OUTPUTS 2
      | CYBER_FAULT (25)
      | Servizi_Informatici_QoS (2)
      mask step_received=|
      | cyber_event=zeros(1,25);
      | cyber_event(1)=Dos_attack;
      | cyber_event(2)=MITM_attack;
      | cyber_event(3)=Virus_Attack;
      | cyber_event(4)=Port_Scan_Attack;
      | cyber_event(5)=BGP_hijacking;
      | cyber_event(6)=BotNet_Attack;
      | cyber_event(7)=Data_Corruption;
      | cyber_event(8)=SW_Change;
      | cyber_event(9)=Config_Change;
      | cyber_event(10)=Port_Saturation;
      | cyber_event(11)=Data_Breach;
      | cyber_event(12)=Unauthorized_Access;
      | cyber_event(13)=Unknown_Device;
      | cyber_event(14)=Congestion_Fault;
      | cyber_event(15)=Interface_Down;
      | cyber_event(16)=Port_Isolation;
      | cyber_event(17)=Rouge_Access;
      | cyber_event(18)=Route_Poisoning;
      | cyber_event(19)=SW_Fault;
      | cyber_event(20)=syslog_adm_login;
      | cyber_event(21)=USB_Device_Insertion;
      | cyber_event(22)=Ransomware;
      | cyber_event(23)=0;
      | cyber_event(24)=0;
      | cyber_event(25)=0;
      |
      | Cyber_Fault=max(CYBER_FAULT, transpose(cyber_event));
      |
      | SW_Fault=max([Virus_Attack Data_Corruption SW_Change] );
      |
      | Service_Fault=1-EXT_SERVICE;
      |
      | Operative_Level=min([(1-Service_Fault) (1-SW_Fault) (1- 0.5 * max(Cyber_Fault))  mean(Reti_QoS)  mean(Sistemi_Informativi_QoS) mean(Servizi_Informatici_QoS)  mean(BENE_ICT_QoS)]);
      |
      | % Il primo elemento rappersenta possibility e si combima
      | % con il max in quanto rende conto del caso migliore
      | % (perche OL)
      |
      | Op_Level2(1)=  min([1-0.3*max(Cyber_Fault) max([use_elem(Reti_QoS,1) use_elem(Sistemi_Informativi_QoS,1) use_elem(Servizi_Informatici_QoS,1) use_elem(BENE_ICT_QoS,1)]) 1-Service_Fault (1-SW_Fault)]);
      |
      | % Il secondo elemento rappersenta necessity e si combima
      | % con il min in quanto rende conto del caso peggiore
      | % (perche OL)
      |
      | Op_Level2(2)= min([1-0.6*max(Cyber_Fault) min([use_elem(Reti_QoS,2) use_elem(Sistemi_Informativi_QoS,2) use_elem(Servizi_Informatici_QoS,2) use_elem(BENE_ICT_QoS,2)]) 1-Service_Fault 1-SW_Fault]);
      |
      | Possibility_Value = Op_Level2(1);
      | Necessity_Value = Op_Level2(2);
      mask step_sended=|
      | CYBER_FAULT=Cyber_Fault;
      |
      | Servizi_Informatici_QoS=Op_Level2;
      mask prompts: Parameter1 "entity name"; Parameter2 "sampling time"; Parameter3 "project"; resources "input resources and state variables"; Parameter10 "Bring state variables to output"; codeupdate "update code from mask"
      mask help: This is a level-2 MATLAB file S-function which demonstrates CISIA entity
      mask DialogControl Container1 Prompt: All parameters
      mask Display: disp('Servizi_Informatici');port_label('input',4,'\color{yellow}\spadesuit','texmode','on');port_label('input',5,'\color{yellow}\spadesuit','texmode','on')
  ADR_Sist_Informativi_1 (508) : M-S-Function  FunctionName=cisia_msfun  Parameters=Parameter1, Parameter2, Parameter3, resources, Parameter10, codeupdate, step_received, step_computed, dynamic_computed, step_sended, id_entity, id_project, id_type, name_type, color  mask(S-function:msfcn_unit_delay){Parameter1='ADR_Sist_Informativi_1', Parameter2=1, Parameter3='Iside', resources=|, Parameter10=off, codeupdate=off, step_received=|, step_computed=, dynamic_computed=, step_sended=|, id_entity=508, id_project=14, id_type=81, name_type=Sistemi_Informativi, color=#59F2F7}
      mask resources=|
      | *** INPUT RESOURCES ***
      | NUM_INPUTS 5
      | CYBER_FAULT (25)
      | Sistemi_Informativi_QoS (2)
      | Reti_QoS (2)
      | Servizi_Informatici_QoS (2)
      | EXT_SERVICE (1)
      |
      | *** STATE VARIABLES ***
      | NUM_VARIABLES 33
      | Operative_Level(NUMERIC)(1)(1)
      | Dos_attack(NUMERIC)(1)(0)
      | MITM_attack(NUMERIC)(1)(0)
      | Virus_Attack(NUMERIC)(1)(0)
      | Port_Scan_Attack(NUMERIC)(1)(0)
      | Cyber_Fault(NUMERIC_ARRAY)(25)(0  0  0  0  0  0  0  0  0  0  0  0  0  0  0  0  0  0  0  0  0  0  0  0  0)
      | BGP_hijacking(NUMERIC)(1)(0)
      | Mechanical_Fault(NUMERIC)(1)(0)
      | Power_Fault(NUMERIC)(1)(0)
      | Unauthorized_Access(NUMERIC)(1)(0)
      | Consumed_Services(NUMERIC_ARRAY)(10)(0  0  0  0  0  0  0  0  0  0)
      | Service_Fault(NUMERIC)(1)(0)
      | BotNet_Attack(NUMERIC)(1)(0)
      | Data_Corruption(NUMERIC)(1)(0)
      | Rouge_Access(NUMERIC)(1)(0)
      | syslog_adm_login(NUMERIC)(1)(0)
      | SW_Change(NUMERIC)(1)(0)
      | Config_Change(NUMERIC)(1)(0)
      | Port_Saturation(NUMERIC)(1)(0)
      | Congestion_Fault(NUMERIC)(1)(0)
      | Route_Poisoning(NUMERIC)(1)(0)
      | Interface_Down(NUMERIC)(1)(0)
      | Port_Isolation(NUMERIC)(1)(0)
      | Unknown_Device(NUMERIC)(1)(0)
      | USB_Device_Insertion(NUMERIC)(1)(0)
      | Computational_Fault(NUMERIC)(1)(0)
      | SW_Fault(NUMERIC)(1)(0)
      | Internal_Cyber_Risk(NUMERIC)(1)(0)
      | Data_Breach(NUMERIC)(1)(0)
      | Ransomware(NUMERIC)(1)(0)
      | Op_Level2(NUMERIC_ARRAY)(2)(0  0)
      | Possibility_Value(NUMERIC)(1)(0)
      | Necessity_Value(NUMERIC)(1)(0)
      |
      | *** OUTPUT RESOURCES ***
      | NUM_OUTPUTS 2
      | CYBER_FAULT (25)
      | Sistemi_Informativi_QoS (2)
      mask step_received=|
      | cyber_event=zeros(1,25);
      | cyber_event(1)=Dos_attack;
      | cyber_event(2)=MITM_attack;
      | cyber_event(3)=Virus_Attack;
      | cyber_event(4)=Port_Scan_Attack;
      | cyber_event(5)=BGP_hijacking;
      | cyber_event(6)=BotNet_Attack;
      | cyber_event(7)=Data_Corruption;
      | cyber_event(8)=SW_Change;
      | cyber_event(9)=Config_Change;
      | cyber_event(10)=Port_Saturation;
      | cyber_event(11)=Data_Breach;
      | cyber_event(12)=Unauthorized_Access;
      | cyber_event(13)=Unknown_Device;
      | cyber_event(14)=Congestion_Fault;
      | cyber_event(15)=Interface_Down;
      | cyber_event(16)=Port_Isolation;
      | cyber_event(17)=Rouge_Access;
      | cyber_event(18)=Route_Poisoning;
      | cyber_event(19)=SW_Fault;
      | cyber_event(20)=syslog_adm_login;
      | cyber_event(21)=USB_Device_Insertion;
      | cyber_event(22)=Ransomware;
      | cyber_event(23)=0;
      | cyber_event(24)=0;
      | cyber_event(25)=0;
      |
      | Cyber_Fault=max(CYBER_FAULT, transpose(cyber_event));
      |
      | Computational_Fault=max([Dos_attack Virus_Attack BotNet_Attack Config_Change Mechanical_Fault] );
      |
      | Service_Fault=1-EXT_SERVICE;
      |
      | Operative_Level=min([(1-Service_Fault) (1-Computational_Fault) (1-0.5*max(Cyber_Fault))  mean(Reti_QoS)  mean(Sistemi_Informativi_QoS)  mean(Servizi_Informatici_QoS)]);
      |
      | % Il primo elemento rappersenta possibility e si combima
      | % con il max in quanto rende conto del caso migliore
      | % (perche OL)
      |
      | Op_Level2(1)=  min([1-0.3*max(Cyber_Fault) max([use_elem(Reti_QoS,1) use_elem(Sistemi_Informativi_QoS,1) use_elem(Servizi_Informatici_QoS,1)]) 1-Service_Fault (1-Computational_Fault)]);
      |
      | % Il secondo elemento rappersenta necessity e si combima
      | % con il min in quanto rende conto del caso peggiore
      | % (perche OL)
      |
      | Op_Level2(2)= min([1-0.6*max(Cyber_Fault) min([use_elem(Reti_QoS,2) use_elem(Sistemi_Informativi_QoS,2) use_elem(Servizi_Informatici_QoS,2)]) 1-Service_Fault 1-Computational_Fault]);
      |
      | Possibility_Value = Op_Level2(1);
      | Necessity_Value = Op_Level2(2);
      mask step_sended=|
      | CYBER_FAULT=Cyber_Fault;
      |
      | Sistemi_Informativi_QoS=Op_Level2;
      mask prompts: Parameter1 "entity name"; Parameter2 "sampling time"; Parameter3 "project"; resources "input resources and state variables"; Parameter10 "Bring state variables to output"; codeupdate "update code from mask"
      mask help: This is a level-2 MATLAB file S-function which demonstrates CISIA entity
      mask DialogControl Container1 Prompt: All parameters
      mask Display: disp('Sistemi_Informativi');port_label('input',1,'\color{yellow}\spadesuit','texmode','on');port_label('input',2,'\color{yellow}\spadesuit','texmode','on');port_label('input',3,'\color{yellow}\spadesuit','texmode','on');port_label('input',4,'\color{yellow}\spadesuit','texmode','on')
  AIR1_org (545) : M-S-Function  FunctionName=cisia_msfun  Parameters=Parameter1, Parameter2, Parameter3, resources, Parameter10, codeupdate, step_received, step_computed, dynamic_computed, step_sended, id_entity, id_project, id_type, name_type, color  mask(S-function:msfcn_unit_delay){Parameter1='AIR1_org', Parameter2=1, Parameter3='Iside', resources=|, Parameter10=off, codeupdate=off, step_received=|, step_computed=, dynamic_computed=, step_sended=|, id_entity=545, id_project=14, id_type=118, name_type=Organization, color=#A2142F}
      mask resources=|
      | *** INPUT RESOURCES ***
      | NUM_INPUTS 6
      | CYBER_FAULT (25)
      | BENE_ICT_QoS (2)
      | FUNZIONI_ESSENZIALI (10)
      | SERVIZI_ESSENZIALI (10)
      | CYBER_RISK (3)
      | PHYSICAL_STRENGTH (1)
      |
      | *** STATE VARIABLES ***
      | NUM_VARIABLES 35
      | Operative_Level(NUMERIC)(1)(1)
      | Dos_attack(NUMERIC)(1)(0)
      | MITM_attack(NUMERIC)(1)(0)
      | Virus_Attack(NUMERIC)(1)(0)
      | Port_Scan_Attack(NUMERIC)(1)(0)
      | Cyber_Fault(NUMERIC_ARRAY)(25)(0  0  0  0  0  0  0  0  0  0  0  0  0  0  0  0  0  0  0  0  0  0  0  0  0)
      | BGP_hijacking(NUMERIC)(1)(0)
      | Mechanical_Fault(NUMERIC)(1)(0)
      | Unauthorized_Access(NUMERIC)(1)(0)
      | Conn_Fault(NUMERIC)(1)(0)
      | BotNet_Attack(NUMERIC)(1)(0)
      | Data_Corruption(NUMERIC)(1)(0)
      | Rouge_Access(NUMERIC)(1)(0)
      | syslog_adm_login(NUMERIC)(1)(0)
      | SW_Change(NUMERIC)(1)(0)
      | Config_Change(NUMERIC)(1)(0)
      | Port_Saturation(NUMERIC)(1)(0)
      | Congestion_Fault(NUMERIC)(1)(0)
      | Physical_Fault(NUMERIC)(1)(0)
      | Route_Poisoning(NUMERIC)(1)(0)
      | Interface_Down(NUMERIC)(1)(0)
      | Port_Isolation(NUMERIC)(1)(0)
      | Unknown_Device(NUMERIC)(1)(0)
      | USB_Device_Insertion(NUMERIC)(1)(0)
      | SW_Fault(NUMERIC)(1)(0)
      | Servizi_Essenziali(NUMERIC_ARRAY)(10)(0  0  0  0  0  0  0  0  0  0)
      | Funzioni_Essenziali(NUMERIC_ARRAY)(10)(0  0  0  0  0  0  0  0  0  0)
      | Internal_Cyber_Risk(NUMERIC)(1)(0)
      | Data_Breach(NUMERIC)(1)(0)
      | availability_fault(NUMERIC)(1)(0)
      | Ransomware(NUMERIC)(1)(0)
      | ExternalCyberFault(NUMERIC_ARRAY)(3)(0  0  0)
      | Op_Level2(NUMERIC_ARRAY)(2)(1  1)
      | Possibility_Value(NUMERIC)(1)(0)
      | Necessity_Value(NUMERIC)(1)(0)
      |
      | *** OUTPUT RESOURCES ***
      | NUM_OUTPUTS 6
      | CYBER_FAULT (25)
      | FUNZIONI_ESSENZIALI (10)
      | SERVIZI_ESSENZIALI (10)
      | CYBER_RISK (3)
      | ORG_QoS (2)
      | EXTERNAL_CYBER_IMPACT (1)
      mask step_received=|
      | cyber_event=zeros(1,25);
      | cyber_event(1)=Dos_attack;
      | cyber_event(2)=MITM_attack;
      | cyber_event(3)=Virus_Attack;
      | cyber_event(4)=Port_Scan_Attack;
      | cyber_event(5)=BGP_hijacking;
      | cyber_event(6)=BotNet_Attack;
      | cyber_event(7)=Data_Corruption;
      | cyber_event(8)=SW_Change;
      | cyber_event(9)=Config_Change;
      | cyber_event(10)=Port_Saturation;
      | cyber_event(11)=Data_Breach;
      | cyber_event(12)=Unauthorized_Access;
      | cyber_event(13)=Unknown_Device;
      | cyber_event(14)=Congestion_Fault;
      | cyber_event(15)=Interface_Down;
      | cyber_event(16)=Port_Isolation;
      | cyber_event(17)=Rouge_Access;
      | cyber_event(18)=Route_Poisoning;
      | cyber_event(19)=SW_Fault;
      | cyber_event(20)=syslog_adm_login;
      | cyber_event(21)=USB_Device_Insertion;
      | cyber_event(22)=Ransomware;
      | cyber_event(23)=0;
      | cyber_event(24)=0;
      | cyber_event(25)=0;
      |
      | Cyber_Fault=max(CYBER_FAULT, transpose(cyber_event));
      |
      |
      | Conn_Fault=max([Dos_attack BGP_hijacking Route_Poisoning Interface_Down Mechanical_Fault] );
      |
      |
      | Servizi_Essenziali=SERVIZI_ESSENZIALI;
      | Funzioni_Essenziali=FUNZIONI_ESSENZIALI;
      |
      | ExternalCyberFault=CYBER_RISK;
      |
      | Operative_Level=min([1-0.5*max(Cyber_Fault) mean(BENE_ICT_QoS) PHYSICAL_STRENGTH]);
      |
      |
      | Physical_Fault=1-PHYSICAL_STRENGTH;
      |
      | % Il primo elemento rappersenta possibility e si combima
      | % con il max in quanto rende conto del caso migliore
      | % (perche OL)
      |
      | Op_Level2(1)=  min([1-0.3*max(Cyber_Fault) BENE_ICT_QoS(1) PHYSICAL_STRENGTH]);
      |
      | % Il secondo elemento rappersenta necessity e si combima
      | % con il min in quanto rende conto del caso peggiore
      | % (perche OL)
      |
      | Op_Level2(2)= min([1-0.6*max(Cyber_Fault) BENE_ICT_QoS(2) PHYSICAL_STRENGTH]);
      |
      | Possibility_Value = Op_Level2(1);
      | Necessity_Value = Op_Level2(2);
      mask step_sended=|
      | SERVIZI_ESSENZIALI=Servizi_Essenziali*(1-Physical_Fault);
      | FUNZIONI_ESSENZIALI=Funzioni_Essenziali*(1-Physical_Fault);
      |
      |
      | ORG_QoS = Op_Level2;
      |
      | % Need to evaluate C-I-A from Cyber_Fault
      | integrity_fault=max([Cyber_Fault(7)  Cyber_Fault(8) Cyber_Fault(22)]);
      |
      | confidentiality_fault=max([Cyber_Fault(2)  Cyber_Fault(3)  Cyber_Fault(6)  Cyber_Fault(9) Cyber_Fault(22)]);
      |
      | availability_fault=max(Cyber_Fault);
      |
      |
      | % C-I-A
      | CYBER_RISK(1)=confidentiality_fault;
      | CYBER_RISK(2)=integrity_fault;
      | CYBER_RISK(3)=availability_fault;
      |
      | % Need to filter the propagable ones
      | CYBER_FAULT = Cyber_Fault;
      |
      |
      | % Need to map from external risks to internal ones
      | EXTERNAL_CYBER_IMPACT=max(ExternalCyberFault);
      mask prompts: Parameter1 "entity name"; Parameter2 "sampling time"; Parameter3 "project"; resources "input resources and state variables"; Parameter10 "Bring state variables to output"; codeupdate "update code from mask"
      mask help: This is a level-2 MATLAB file S-function which demonstrates CISIA entity
      mask DialogControl Container1 Prompt: All parameters
      mask Display: disp('Organization')
  CIA_pers (513) : M-S-Function  FunctionName=cisia_msfun  Parameters=Parameter1, Parameter2, Parameter3, resources, Parameter10, codeupdate, step_received, step_computed, dynamic_computed, step_sended, id_entity, id_project, id_type, name_type, color  mask(S-function:msfcn_unit_delay){Parameter1='CIA_pers', Parameter2=1, Parameter3='Iside', resources=|, Parameter10=off, codeupdate=off, step_received=Operative_Level = 1;, step_computed=, dynamic_computed=, step_sended=PERSONALE_QoS = Operative_Level;, id_entity=513, id_project=14, id_type=88, name_type=personale, color=#E2F029}
      mask resources=|
      | *** INPUT RESOURCES ***
      | NUM_INPUTS 0
      |
      | *** STATE VARIABLES ***
      | NUM_VARIABLES 1
      | Operative_Level(NUMERIC)(1)(1)
      |
      | *** OUTPUT RESOURCES ***
      | NUM_OUTPUTS 1
      | PERSONALE_QoS (1)
      mask prompts: Parameter1 "entity name"; Parameter2 "sampling time"; Parameter3 "project"; resources "input resources and state variables"; Parameter10 "Bring state variables to output"; codeupdate "update code from mask"
      mask help: This is a level-2 MATLAB file S-function which demonstrates CISIA entity
      mask DialogControl Container1 Prompt: All parameters
      mask Display: disp('personale')
  FCO_pers (383) : M-S-Function  FunctionName=cisia_msfun  Parameters=Parameter1, Parameter2, Parameter3, resources, Parameter10, codeupdate, step_received, step_computed, dynamic_computed, step_sended, id_entity, id_project, id_type, name_type, color  mask(S-function:msfcn_unit_delay){Parameter1='FCO_pers', Parameter2=1, Parameter3='Iside', resources=|, Parameter10=off, codeupdate=off, step_received=Operative_Level = 1;, step_computed=, dynamic_computed=, step_sended=PERSONALE_QoS = Operative_Level;, id_entity=383, id_project=14, id_type=88, name_type=personale, color=#E2F029}
      mask resources=|
      | *** INPUT RESOURCES ***
      | NUM_INPUTS 0
      |
      | *** STATE VARIABLES ***
      | NUM_VARIABLES 1
      | Operative_Level(NUMERIC)(1)(1)
      |
      | *** OUTPUT RESOURCES ***
      | NUM_OUTPUTS 1
      | PERSONALE_QoS (1)
      mask prompts: Parameter1 "entity name"; Parameter2 "sampling time"; Parameter3 "project"; resources "input resources and state variables"; Parameter10 "Bring state variables to output"; codeupdate "update code from mask"
      mask help: This is a level-2 MATLAB file S-function which demonstrates CISIA entity
      mask DialogControl Container1 Prompt: All parameters
      mask Display: disp('personale')
  Goto5 : Goto  Commented=on  GotoTag=SERVIZI_GOV1
  MinMax{2..4,6,8} (5 alike) : MinMax  Function=max  Inputs=2
  MinMax7 : MinMax  Function=max  Inputs=3
  Subsystem1 : Subsystem  mask{num_serv=1, operation1=All services required, operation2=All providers required, out_service=none, consumed1=[1 0 0 0 0 0 0 0 0 0]}
      mask prompts: num_serv "Providers in input"; operation1 "For each single service provider"; operation2 "Among providers"; out_service "Vectorial output"; consumed1 "Required 1"
      mask TypeOptions num_serv: 1
      mask TypeOptions operation1: All services required | At least one
      mask TypeOptions operation2: All providers required
      mask TypeOptions out_service: none | S1 | S2 | S3 | S4 | S5 | S6 | S7 | S8 | S9 | S10 | F1 | F2 | F3 | F4 | F5 | F6 | F7 | F8 | F9 | F10
  Subsystem10 : Subsystem  mask{num_serv=1, operation1=All services required, operation2=All providers required, out_service=S2, consumed1=[1 0 0 0 0 0 0 0 0 0]}
      mask prompts: num_serv "Providers in input"; operation1 "For each single service provider"; operation2 "Among providers"; out_service "Vectorial output"; consumed1 "Required 1"
      mask TypeOptions num_serv: 1
      mask TypeOptions operation1: All services required | At least one
      mask TypeOptions operation2: All providers required
      mask TypeOptions out_service: none | S1 | S2 | S3 | S4 | S5 | S6 | S7 | S8 | S9 | S10 | F1 | F2 | F3 | F4 | F5 | F6 | F7 | F8 | F9 | F10
  Subsystem3 : Subsystem  mask{num_serv=1, operation1=All services required, operation2=All providers required, out_service=none, consumed1=[1 0 0 0 0 0 0 0 0 0]}
      mask prompts: num_serv "Providers in input"; operation1 "For each single service provider"; operation2 "Among providers"; out_service "Vectorial output"; consumed1 "Required 1"
      mask TypeOptions num_serv: 1
      mask TypeOptions operation1: All services required | At least one
      mask TypeOptions operation2: All providers required
      mask TypeOptions out_service: none | S1 | S2 | S3 | S4 | S5 | S6 | S7 | S8 | S9 | S10 | F1 | F2 | F3 | F4 | F5 | F6 | F7 | F8 | F9 | F10
  Subsystem4 : Subsystem  mask{num_serv=1, operation1=All services required, operation2=All providers required, out_service=S1, consumed1=[1 0 0 0 0 0 0 0 0 0]}
      mask prompts: num_serv "Providers in input"; operation1 "For each single service provider"; operation2 "Among providers"; out_service "Vectorial output"; consumed1 "Required 1"
      mask TypeOptions num_serv: 1
      mask TypeOptions operation1: All services required | At least one
      mask TypeOptions operation2: All providers required
      mask TypeOptions out_service: none | S1 | S2 | S3 | S4 | S5 | S6 | S7 | S8 | S9 | S10 | F1 | F2 | F3 | F4 | F5 | F6 | F7 | F8 | F9 | F10
  Subsystem5 : Subsystem  mask{num_serv=1, operation1=All services required, operation2=All providers required, out_service=none, consumed1=[0 0 1 0 0 0 0 0 0 0]}
      mask prompts: num_serv "Providers in input"; operation1 "For each single service provider"; operation2 "Among providers"; out_service "Vectorial output"; consumed1 "Required 1"
      mask TypeOptions num_serv: 1
      mask TypeOptions operation1: All services required | At least one
      mask TypeOptions operation2: All providers required
      mask TypeOptions out_service: none | S1 | S2 | S3 | S4 | S5 | S6 | S7 | S8 | S9 | S10 | F1 | F2 | F3 | F4 | F5 | F6 | F7 | F8 | F9 | F10
  Subsystem6 : Subsystem  mask{num_serv=1, operation1=All services required, operation2=All providers required, out_service=none, consumed1=[1 0 0 0 0 0 0 0 0 0]}
      mask prompts: num_serv "Providers in input"; operation1 "For each single service provider"; operation2 "Among providers"; out_service "Vectorial output"; consumed1 "Required 1"
      mask TypeOptions num_serv: 1
      mask TypeOptions operation1: All services required | At least one
      mask TypeOptions operation2: All providers required
      mask TypeOptions out_service: none | S1 | S2 | S3 | S4 | S5 | S6 | S7 | S8 | S9 | S10 | F1 | F2 | F3 | F4 | F5 | F6 | F7 | F8 | F9 | F10
  Subsystem7 : Subsystem  mask{num_serv=1, operation1=All services required, operation2=All providers required, out_service=none, consumed1=[0 0 1 0 0 0 0 0 0 0]}
      mask prompts: num_serv "Providers in input"; operation1 "For each single service provider"; operation2 "Among providers"; out_service "Vectorial output"; consumed1 "Required 1"
      mask TypeOptions num_serv: 1
      mask TypeOptions operation1: All services required | At least one
      mask TypeOptions operation2: All providers required
      mask TypeOptions out_service: none | S1 | S2 | S3 | S4 | S5 | S6 | S7 | S8 | S9 | S10 | F1 | F2 | F3 | F4 | F5 | F6 | F7 | F8 | F9 | F10
  Subsystem8 : Subsystem  mask{num_serv=1, operation1=All services required, operation2=All providers required, out_service=none, consumed1=[1 0 0 0 0 0 0 0 0 0]}
      mask prompts: num_serv "Providers in input"; operation1 "For each single service provider"; operation2 "Among providers"; out_service "Vectorial output"; consumed1 "Required 1"
      mask TypeOptions num_serv: 1
      mask TypeOptions operation1: All services required | At least one
      mask TypeOptions operation2: All providers required
      mask TypeOptions out_service: none | S1 | S2 | S3 | S4 | S5 | S6 | S7 | S8 | S9 | S10 | F1 | F2 | F3 | F4 | F5 | F6 | F7 | F8 | F9 | F10
  Subsystem9 : Subsystem  mask{num_serv=1, operation1=All services required, operation2=All providers required, out_service=S3, consumed1=[0 1 0 0 0 0 0 0 0 0]}
      mask prompts: num_serv "Providers in input"; operation1 "For each single service provider"; operation2 "Among providers"; out_service "Vectorial output"; consumed1 "Required 1"
      mask TypeOptions num_serv: 1
      mask TypeOptions operation1: All services required | At least one
      mask TypeOptions operation2: All providers required
      mask TypeOptions out_service: none | S1 | S2 | S3 | S4 | S5 | S6 | S7 | S8 | S9 | S10 | F1 | F2 | F3 | F4 | F5 | F6 | F7 | F8 | F9 | F10
  delay : Subsystem  mask{delay=0.9, output=ones(1,10)}
  delay1 : Subsystem  mask{delay=0.9, output=ones(1,10)}
  maxmin : MATLAB Function  TreatAsAtomicUnit=on
  maxmin1 : MATLAB Function  TreatAsAtomicUnit=on
  CYBER_FAULT : Outport
  FUNZIONI_AIR1 : Outport  Port=2
  SERVIZI_AIR1 : Outport  Port=3
  CYBER_RISK_AIR1 : Outport  Port=4
  AIR1_QoS : Outport  Port=5
  EXTERNAL_CYBER_IMPACT : Outport  Port=6
  wires:
  AIR1_org (545)/1 -> CYBER_FAULT/1  "CYBER_FAULT"
  AIR1_org (545)/2 -> delay/1(in)  "FUNZIONI_ESSENZIALI"
  AIR1_org (545)/3 -> delay1/1(in)  "SERVIZI_ESSENZIALI"
  ADR_BeneICT_1 (505)/3 -> MinMax3/1  "FUNZIONI_ESSENZIALI"
  MinMax4/1 -> AIR1_org (545)/1  "CYBER_FAULT"
  ADR_BeneICT_2 (506)/1 -> MinMax4/2  "CYBER_FAULT"
  ADR_BeneICT_1 (505)/2 -> maxmin1/2(u2)  "BENE_ICT_QoS"
  ADR_Physical/1(Physical) -> AIR1_org (545)/6  "PHYSICAL_STRENGTH"
  ADR_BeneICT_2 (506)/3 -> MinMax3/2  "FUNZIONI_ESSENZIALI"
  maxmin1/1(y) -> AIR1_org (545)/2  "BENE_ICT_QoS"
  ADR_Aeroporto_FCO (399)/1 -> ADR_Rete_1 (509)/1  "CYBER_FAULT"
  ADR_BeneICT_2 (506)/2 -> maxmin1/1(u1)  "BENE_ICT_QoS"
  ADR_BeneICT_1 (505)/1 -> MinMax4/1  "CYBER_FAULT"
  ADR_Rete_1 (509)/1 -> MinMax7/1  "CYBER_FAULT"
  FCO_pers (383)/1 -> ADR_Aeroporto_FCO (399)/2  "PERSONALE_QoS"
  CYBER_RISK_TELCO1/1 -> [CYBER_RISK_TELCO1]
  SERVIZI_TELCO1/1 -> [SERVIZI_TELCO1]
  SERVIZI_ELE1/1 -> [SERVIZI_ELE1]
  SERVIZI_ELE2/1 -> [SERVIZI_ELE2]
  CIA_pers (513)/1 -> ADR_Aeroporto_CIA (512)/2  "PERSONALE_QoS"
  Subsystem5/1(EXT) -> ADR_Aeroporto_CIA (512)/4  "SERVIZI_Connessione"
  maxmin/1(y) -> ADR_Rete_2 (510)/3  "NODO_CYBER_QoS"
  ADR_Aeroporto_CIA (512)/1 -> MinMax7/3  "CYBER_FAULT"
  ADR_Rete_1 (509)/2 -> ADR_Rete_2 (510)/2  "Reti_QoS"
  Subsystem3/1(EXT) -> ADR_Sist_Informativi_1 (508)/5  "EXT_SERVICE"
  [SERVIZI_ELE1] -> Subsystem3/1(servizio)
  Subsystem1/1(EXT) -> ADR_Serv_Informatico_1 (507)/6  "EXT_SERVICE"
  [SERVIZI_ELE1] -> Subsystem1/1(servizio)
  MinMax8/1 -> ADR_BeneICT_2 (506)/6  "SERVIZIO_ESTERNO"
  [SERVIZI_TELCO1] -> Subsystem10/1(servizio)
  Subsystem4/2(EXT_V) -> ADR_BeneICT_1 (505)/6  "SERVIZIO_ESTERNO"
  [SERVIZI_TELCO1] -> Subsystem4/1(servizio)
  ADR_Serv_Informatico_1 (507)/1 -> ADR_BeneICT_2 (506)/1, ADR_BeneICT_1 (505)/1  "CYBER_FAULT"
  ADR_Sist_Informativi_1 (508)/2 -> ADR_Serv_Informatico_1 (507)/2  "Sistemi_Informativi_QoS"
  ADR_Rete_2 (510)/2 -> ADR_Serv_Informatico_1 (507)/3  "Reti_QoS"
  MinMax2/1 -> ADR_Serv_Informatico_1 (507)/1  "CYBER_FAULT"
  ADR_Rete_2 (510)/1 -> MinMax2/2  "CYBER_FAULT"
  ADR_Sist_Informativi_1 (508)/1 -> MinMax2/1  "CYBER_FAULT"
  ADR_Serv_Informatico_1 (507)/2 -> ADR_BeneICT_2 (506)/4, ADR_BeneICT_1 (505)/4  "Servizi_Informatici_QoS"
  ADR_BeneICT_1 (505)/4 -> MinMax6/1  "SERVIZI_ESSENZIALI"
  ADR_BeneICT_2 (506)/4 -> MinMax6/2  "SERVIZI_ESSENZIALI"
  MinMax6/1 -> AIR1_org (545)/4  "SERVIZI_ESSENZIALI"
  MinMax3/1 -> AIR1_org (545)/3  "FUNZIONI_ESSENZIALI"
  delay/1(out) -> FUNZIONI_AIR1/1
  [CYBER_RISK_TELCO1] -> AIR1_org (545)/5  "CYBER_RISK"
  ADR_Nodo_1 (511)/2 -> maxmin/1(u1)  "NODO_CYBER_QoS"
  MinMax7/1 -> ADR_Rete_2 (510)/1  "CYBER_FAULT"
  ADR_Nodo_1 (511)/1 -> MinMax7/2  "CYBER_FAULT"
  [SERVIZI_TELCO1] -> Subsystem5/1(servizio)  "SERVIZI_Connessione"
  Subsystem6/1(EXT) -> ADR_Aeroporto_CIA (512)/3  "SERVIZI_Elettrici"
  [SERVIZI_ELE2] -> Subsystem6/1(servizio)  "SERVIZI_ELETTRICI"
  Subsystem7/1(EXT) -> ADR_Aeroporto_FCO (399)/4  "SERVIZI_Connessione"
  Subsystem8/1(EXT) -> ADR_Aeroporto_FCO (399)/3  "SERVIZI_Elettrici"
  [SERVIZI_ELE1] -> Subsystem8/1(servizio)  "SERVIZI_ELETTRICI"
  [SERVIZI_TELCO1] -> Subsystem7/1(servizio)  "SERVIZI_Connessione"
  ADR_Aeroporto_CIA (512)/3 -> ADR_Physical/2(N2)  "NODO_PHISICAL_QoS"
  ADR_Aeroporto_CIA (512)/2 -> maxmin/2(u2)  "NODO_CYBER_QoS"
  ADR_Aeroporto_FCO (399)/3 -> ADR_Physical/1(N1)  "NODO_PHISICAL_QoS"
  ADR_Aeroporto_FCO (399)/2 -> ADR_Rete_1 (509)/3  "NODO_CYBER_QoS"
  SERVIZI_BANK1/1 -> [SERVIZI_BANK1]
  [SERVIZI_BANK1] -> Subsystem9/1(servizio)
  Subsystem10/2(EXT_V) -> MinMax8/1  "SERVIZIO_ESTERNO"
  Subsystem9/2(EXT_V) -> MinMax8/2  "SERVIZIO_ESTERNO"
  SERVIZI_GOV1/1 -> Goto5/1
  delay1/1(out) -> SERVIZI_AIR1/1
  AIR1_org (545)/4 -> CYBER_RISK_AIR1/1  "CYBER_RISK"
  AIR1_org (545)/5 -> AIR1_QoS/1  "ORG_QoS"
  AIR1_org (545)/6 -> EXTERNAL_CYBER_IMPACT/1  "EXTERNAL_CYBER_IMPACT"
